simulink model "SimPara_DTDSM_2b_2or_512osr"  (R2019b)
settings: Solver=VariableStepAuto  StartTime=0.0  StopTime=ts*(Mpoints+10)  RelTol=1e-3
InitFcn:
  | %fs=256*2e4;
  | %osr=512;
  | ts=1/fs;
  | 
  | Ncycle=37;
  | Mpoints=2^16;
  | fin=fs*Ncycle/Mpoints;
  | 
  | 
  | ref=4/3;
values from neighbouring files (symbols this model uses):
  fs = osr*2e4    (= 10240000)    [CTSDM.m]
  osr = 512    [CTSDM.m]    (also in ENOB.m = logspace(log10(64), log10(2^15), 1000); SNR.m = logspace(log10(64), log10(2^15), 1000))
undefined symbols (not defined in the file or in its folder): argo
libraries: SDtoolbox x4
settings Model: Creator=lenovo  LastModifiedBy=lenovo

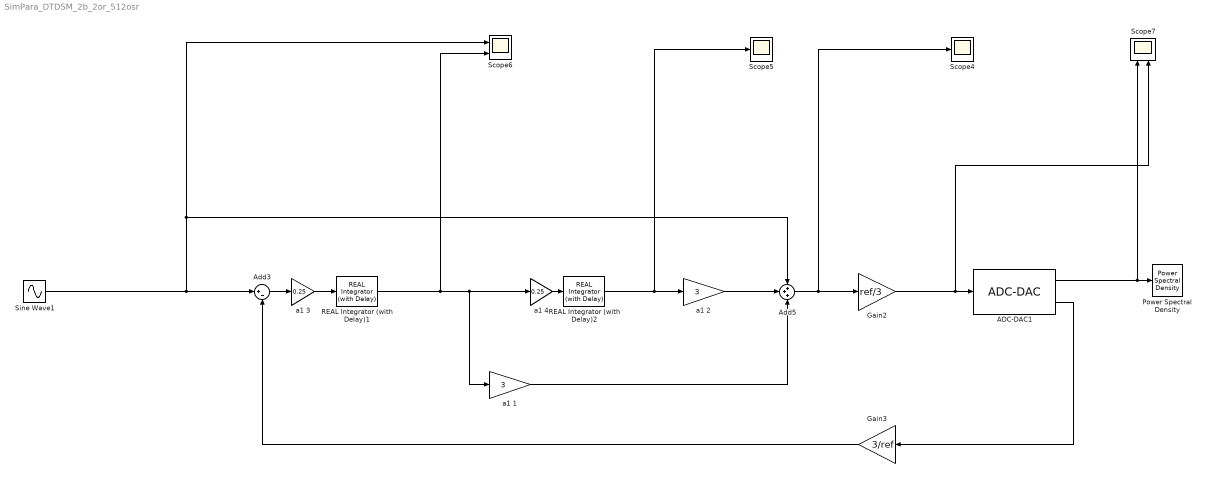
== system SimPara_DTDSM_2b_2or_512osr ==
  ADC-DAC1 : SDtoolbox/ADC-DAC  k=3  MM=off  match=0  CST=0  VVG=off  argo=argo(:,3)  LF=on  NF=retA.log
      settings: SourceProductName=SDtoolbox
  Add3 : Sum  Inputs=|+-
  Add5 : Sum  Inputs=+++
  Gain2 : Gain  Gain=ref/3
  Gain3 : Gain  Gain=3/ref
  Power Spectral Density : SDtoolbox/Power Spectral Density  SN=2  Fs=fs  fBL=1  fBH=fs/(2*osr)  Fin=fin  N=Mpoints  Ntransient=10  VW=on  savename=110  Scale_type=logarithmic
      settings: SourceProductName=SDtoolbox
  REAL Integrator (with Delay)1 : SDtoolbox/REAL Integrator (with Delay)  Ts=ts  alfa=(10^4-1)/10^4  Amax=3.3  sr=200e6  GBW=2e8
      settings: SourceProductName=SDtoolbox
  REAL Integrator (with Delay)2 : SDtoolbox/REAL Integrator (with Delay)  Ts=ts  alfa=(10^4-1)/10^4  Amax=3.3  sr=200e6  GBW=2e8
      settings: SourceProductName=SDtoolbox
  Scope4 : Scope
  Scope5 : Scope
  Scope6 : Scope  NumInputPorts=2
  Scope7 : Scope  NumInputPorts=2
  Sine Wave1 : Sin  Amplitude=2.1  Frequency=fin*2*pi  SampleTime=ts
  a1 1 : Gain  Gain=3
  a1 2 : Gain  Gain=3
  a1 3 : Gain  Gain=0.25
  a1 4 : Gain  Gain=0.25
  wires:
  Add5/1 -> Scope4/1, Gain2/1
  Gain2/1 -> ADC-DAC1/1, Scope7/2
  ADC-DAC1/2 -> Gain3/1
  REAL Integrator (with Delay)2/1 -> a1 2/1, Scope5/1
  a1 1/1 -> Add5/3
  ADC-DAC1/1 -> Power Spectral Density/1, Scope7/1
  REAL Integrator (with Delay)1/1 -> Scope6/2, a1 4/1, a1 1/1
  Sine Wave1/1 -> Add3/1, Add5/1, Scope6/1
  Gain3/1 -> Add3/2
  a1 2/1 -> Add5/2
  a1 3/1 -> REAL Integrator (with Delay)1/1
  Add3/1 -> a1 3/1
  a1 4/1 -> REAL Integrator (with Delay)2/1
